simulink library "csc_snp_sensor_prep_mtv_lib"  (R2014b)
settings: Solver=ode45  SolverMode=SingleTasking  StartTime=0.0  StopTime=10.0  RelTol=1e-3
undefined symbols (not defined in the file or in its folder): kfl_topo_z_to_alt, snp_meas_noise_alt, snp_meas_noise_indep, snp_R_lower_limit_alt, snp_zero_index, snp_zero_meas
libraries: util_info_lib x1, csc_hmg_homoraphy_meas_lib x1, csc_imu_sensor_prep_mtv_lib x1, csc_rsp_radar_sensor_prep_lib x1, csc_stg_tracker_sensor_prep_lib x1, csu_egm_estimated_gravity_model_mtv_lib x1, csu_rgm_rtk_gps_meas_lib x1, util_quat_lib x1
settings Model: ExtModeAutoUpdateStatusClock=off  Creator=Administrator  LastModifiedBy=mstewart

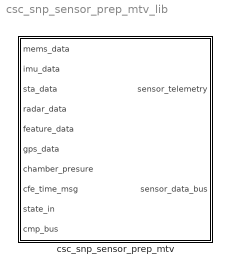
== system csc_snp_sensor_prep_mtv_lib ==
  csc_snp_sensor_prep_mtv : Subsystem

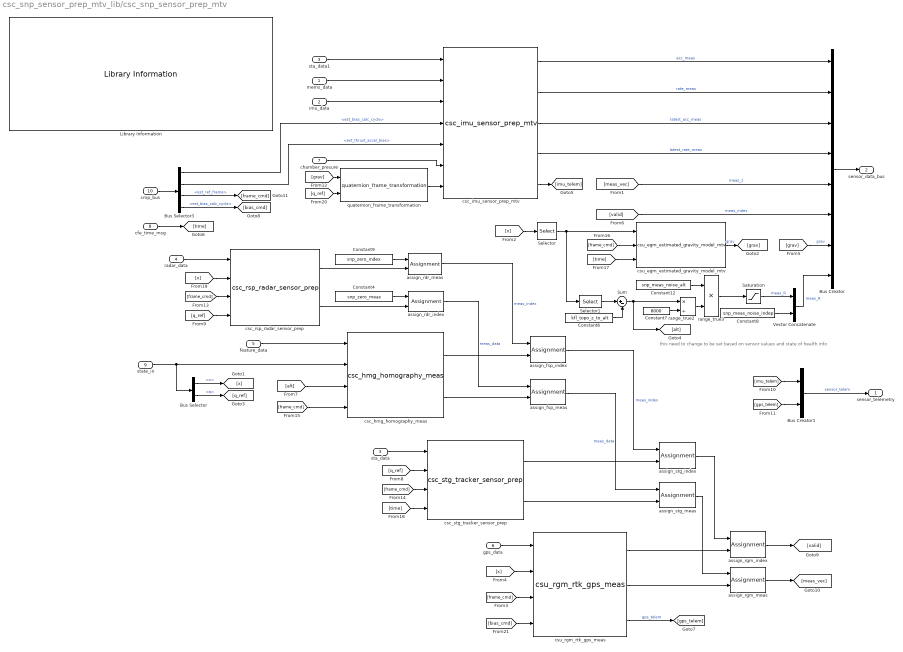
== system csc_snp_sensor_prep_mtv_lib/csc_snp_sensor_prep_mtv ==
  note: this need to change to be set based on sensor values and state of health info
  mems_data : Inport
  imu_data : Inport  Port=2
  sta_data : Inport  Port=3
  radar_data : Inport  Port=4
  feature_data : Inport  Port=5
  gps_data : Inport  Port=6
  chamber_presure : Inport  Port=7
  cfe_time_msg : Inport  Port=8
  state_in : Inport  Port=9
  cmp_bus : Inport  Port=10
  Bus Creator : BusCreator  Inputs=8
  Bus Creator1 : BusCreator  Inputs=2
  Bus Selector : BusSelector  OutputSignals=x,q
  Bus Selector3 : BusSelector  OutputSignals=est_bias_calc_cycle,est_thrust_accel_bias,est_ref_frame,est_bias_calc_cycle
  Constant12 : Constant  Value=snp_meas_noise_alt
  Constant4 : Constant  Value=snp_zero_meas
  Constant6 : Constant  Value=kfl_topo_z_to_alt
  Constant7 : Constant  Value=8000
  Constant8 : Constant  Value=snp_meas_noise_indep
  Constant9 : Constant  Value=snp_zero_index
  Library Information : util_info_lib/Library Information  owner='NONE'
  Saturation : Saturate  UpperLimit=1e20*[1 1 1]  LowerLimit=snp_R_lower_limit_alt
  Selector : Selector  InputPortWidth=kfl_n_state  Indices=kfl_pos_index
  Selector1 : Selector  InputPortWidth=3  Indices=[3]
  Sum : Sum  Inputs=|+-
  Vector Concatenate : Concatenate
  assign_fsp_index : Assignment  Indices=snp_fsp_index
  assign_fsp_meas : Assignment  Indices=snp_fsp_index
  assign_rdr_index : Assignment  Indices=snp_rdr_index
  assign_rdr_meas : Assignment  Indices=snp_rdr_index
  assign_rgm_index : Assignment  Indices=snp_rgm_index
  assign_rgm_meas : Assignment  Indices=snp_rgm_index
  assign_stg_index : Assignment  Indices=snp_stg_index
  assign_stg_meas : Assignment  Indices=snp_stg_index
  csc_hmg_homography_meas : csc_hmg_homoraphy_meas_lib/csc_hmg_homography_meas
  csc_imu_sensor_prep_mtv : csc_imu_sensor_prep_mtv_lib/csc_imu_sensor_prep_mtv
  csc_rsp_radar_sensor_prep : csc_rsp_radar_sensor_prep_lib/csc_rsp_radar_sensor_prep
  csc_stg_tracker_sensor_prep : csc_stg_tracker_sensor_prep_lib/csc_stg_tracker_sensor_prep
  csu_egm_estimated_gravity_model_mtv : csu_egm_estimated_gravity_model_mtv_lib/csu_egm_estimated_gravity_model_mtv
  csu_rgm_rtk_gps_meas : csu_rgm_rtk_gps_meas_lib/csu_rgm_rtk_gps_meas
  quaternion_frame_transformation : util_quat_lib/quaternion_frame_transformation  SystemSampleTime=-1
  range_true2 : Product  Inputs=*/  RndMeth=Zero
  range_true3 : Product  RndMeth=Zero
  sta_data1 : InportShadow  Port=3
  sensor_telemetry : Outport
  sensor_data_bus : Outport  Port=2
  wires:
  imu_data/1 -> csc_imu_sensor_prep_mtv/3
  Bus Selector3/2 -> csc_imu_sensor_prep_mtv/5  "<est_thrust_accel_bias>"
  chamber_presure/1 -> csc_imu_sensor_prep_mtv/6
  [bias_cmd] -> csu_rgm_rtk_gps_meas/4
  Bus Selector3/4 -> [bias_cmd]  "<est_bias_calc_cycle>"
  [q_ref] -> quaternion_frame_transformation/2
  quaternion_frame_transformation/1 -> csc_imu_sensor_prep_mtv/7
  [grav] -> quaternion_frame_transformation/1
  csu_egm_estimated_gravity_model_mtv/1 -> [grav]  "grav"
  Bus Selector3/1 -> csc_imu_sensor_prep_mtv/4  "<est_bias_calc_cycle>"
  csu_rgm_rtk_gps_meas/3 -> [gps_telem]  "gps_telem"
  [gps_telem] -> Bus Creator1/2
  [imu_telem] -> Bus Creator1/1
  csc_imu_sensor_prep_mtv/5 -> [imu_telem]
  Bus Creator1/1 -> sensor_telemetry/1  "sensor_telem"
  assign_rgm_meas/1 -> [meas_vec]
  assign_rgm_index/1 -> [valid]
  csu_rgm_rtk_gps_meas/2 -> assign_rgm_meas/2
  csu_rgm_rtk_gps_meas/1 -> assign_rgm_index/2
  [x] -> csu_rgm_rtk_gps_meas/2
  [frame_cmd] -> csu_rgm_rtk_gps_meas/3
  gps_data/1 -> csu_rgm_rtk_gps_meas/1
  mems_data/1 -> csc_imu_sensor_prep_mtv/2
  sta_data1/1 -> csc_imu_sensor_prep_mtv/1
  csc_imu_sensor_prep_mtv/4 -> Bus Creator/4  "latest_rate_meas"
  csc_imu_sensor_prep_mtv/3 -> Bus Creator/3  "latest_acc_meas"
  csc_imu_sensor_prep_mtv/2 -> Bus Creator/2  "rate_meas"
  csc_imu_sensor_prep_mtv/1 -> Bus Creator/1  "acc_meas"
  csc_hmg_homography_meas/1 -> assign_fsp_index/2
  [q_ref] -> csc_rsp_radar_sensor_prep/4
  [alt] -> csc_hmg_homography_meas/3
  Constant9/1 -> assign_rdr_meas/1
  Constant4/1 -> assign_rdr_index/1
  csc_rsp_radar_sensor_prep/2 -> assign_rdr_index/2
  feature_data/1 -> csc_hmg_homography_meas/1
  [valid] -> Bus Creator/6  "meas_index"
  assign_rdr_meas/1 -> assign_fsp_index/1  "meas_index"
  assign_rdr_index/1 -> assign_fsp_meas/1  "meas_data"
  csc_hmg_homography_meas/2 -> assign_fsp_meas/2
  Bus Selector/1 -> [x]  "<x>"
  [x] -> Selector/1
  state_in/1 -> csc_hmg_homography_meas/2, Bus Selector/1
  [grav] -> Bus Creator/7  "grav"
  [meas_vec] -> Bus Creator/5  "meas_z"
  radar_data/1 -> csc_rsp_radar_sensor_prep/1
  csc_rsp_radar_sensor_prep/1 -> assign_rdr_meas/2
  Bus Creator/1 -> sensor_data_bus/1
  Selector/1 -> csu_egm_estimated_gravity_model_mtv/1, Selector1/1
  Constant6/1 -> Sum/2
  Selector1/1 -> Sum/1
  range_true2/1 -> range_true3/2
  Constant12/1 -> range_true3/1
  range_true3/1 -> Saturation/1
  cfe_time_msg/1 -> [time]
  Sum/1 -> range_true2/1, [alt]
  Constant7/1 -> range_true2/2
  sta_data/1 -> csc_stg_tracker_sensor_prep/1
  Bus Selector/2 -> [q_ref]  "<q>"
  [q_ref] -> csc_stg_tracker_sensor_prep/2
  [x] -> csc_rsp_radar_sensor_prep/2
  assign_fsp_index/1 -> assign_stg_index/1  "meas_index"
  assign_stg_index/1 -> assign_rgm_index/1
  assign_stg_meas/1 -> assign_rgm_meas/1
  assign_fsp_meas/1 -> assign_stg_meas/1  "meas_data"
  csc_stg_tracker_sensor_prep/2 -> assign_stg_meas/2
  csc_stg_tracker_sensor_prep/1 -> assign_stg_index/2
  cmp_bus/1 -> Bus Selector3/1
  [frame_cmd] -> csc_rsp_radar_sensor_prep/3
  [frame_cmd] -> csc_stg_tracker_sensor_prep/3
  [frame_cmd] -> csc_hmg_homography_meas/4
  [frame_cmd] -> csu_egm_estimated_gravity_model_mtv/2
  [time] -> csu_egm_estimated_gravity_model_mtv/3
  Bus Selector3/3 -> [frame_cmd]  "<est_ref_frame>"
  Saturation/1 -> Vector Concatenate/1  "meas_R"
  Vector Concatenate/1 -> Bus Creator/8  "meas_R"
  Constant8/1 -> Vector Concatenate/2
  [time] -> csc_stg_tracker_sensor_prep/4
